simulink model "TP1_SIM_R3FOC_ctrl"  (R2023b)
settings: Solver=ode15s  StartTime=0.0  StopTime=0.2  FixedStep=1e-6  RelTol=1e-5  EnableMultiTasking=on
values from neighbouring files (symbols this model uses):
  deltat = deltat_2    (= 35)    [tp1_b.m]
  theta = 3    [tp1_b.m]
libraries: spsThyristorLib x6, spsNeutralLib x5, spsVoltageMeasurementLib x4, spsMeanLib x3, spsCurrentMeasurementLib x1, spsGroundLib x1, spsSeriesRLCLoadLib x1, spsThreePhaseProgrammableVoltageSourceLib x1, spspowerguiLib x1
settings Model: Creator=Monina  LastModifiedBy=Amadeo
settings SolverCC: AlgebraicLoopSolver=TrustRegion
settings DataIOCC: SaveFormat=Array  SignalLoggingSaveFormat=ModelDataLogs  ReturnWorkspaceOutputs=off
settings OptimizationCC: ExpressionDepthLimit=2147483647  LifeSpan=inf
settings DebuggingCC: UnderspecifiedInitializationDetection=Classic  MergeDetectMultiDrivingBlocksExec=none  SolverPrmCheckMsg=warning  FcnCallInpInsideContextMsg=warning  UnconnectedInputMsg=warning  UnconnectedOutputMsg=warning  UnconnectedLineMsg=warning  StateNameClashWarn=warning  SFUnexpectedBacktrackingDiag=warning  SFNoUnconditionalDefaultTransitionDiag=warning  SFExecutionAtInitializationDiag=none  ArithmeticOperatorsInVariantConditions=warning
settings HardwareCC: ProdBitPerPointer=32  ProdBitPerSizeT=32  ProdBitPerPtrDiffT=32  ProdLargestAtomicFloat=None  ProdIntDivRoundTo=Undefined  ProdEndianess=Unspecified  ProdWordSize=32  ProdHWDeviceType=32-bit Generic
settings ModelReferenceCC: EnableRefExpFcnMdlSchedulingChecks=on  PropagateSignalLabelsOutOfModel=off
settings SFSimCC: SimUseLocalCustomCode=off  CustomCodeUndefinedFunction=UseInterfaceOnly
settings RTWCC: RTWUseLocalCustomCode=off
settings CodeAppCC: StateflowObjectComments=on
settings GRTTargetCC: TargetLangStandard=C89/C90 (ANSI)  CombineOutputUpdateFcns=off  GRTInterface=on
settings ConfigComp: CovMetricSettings=dw  CovSaveCumulativeToWorkspaceVar=on  CovSaveSingleToWorkspaceVar=on  CovExternalEMLEnable=off  CovSFcnEnable=off
settings SimscapeCC: SimscapeNormalizeSystem=off

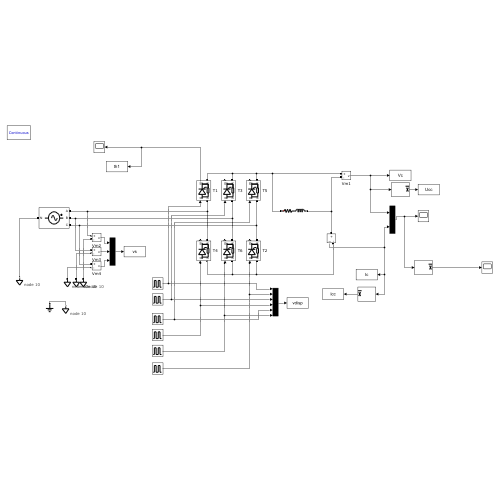
[thumbnail: Simulink's stored preview of the top-level diagram]
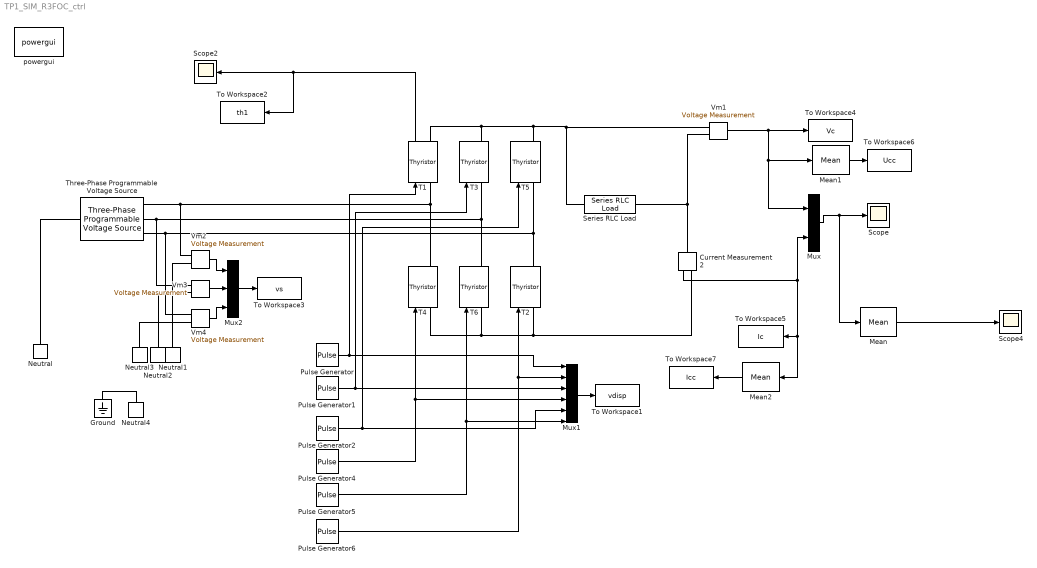
== system TP1_SIM_R3FOC_ctrl ==
  Current Measurement2 : spsCurrentMeasurementLib/Current Measurement  PhasorSimulation=off  OutputType=Complex  PSBequivalent=0
  Ground : spsGroundLib/Ground  LConnTagsString=a
  Mean : spsMeanLib/Mean  Freq=50  Vinit=0  Ts=0
  Mean1 : spsMeanLib/Mean  Freq=50  Vinit=0  Ts=0
  Mean2 : spsMeanLib/Mean  Freq=50  Vinit=0  Ts=0
  Mux : Mux  Inputs=2
  Mux1 : Mux  Inputs=6
  Mux2 : Mux  Inputs=3
  Neutral{,1..4} (5 alike) : spsNeutralLib/Neutral  LConnTagsString=a  NodeNumber=10
      settings: AttributesFormatString=node %<NodeNumber>  LibrarySourceBlock=sps_lib/Utilities/Neutral
  Pulse Generator : DiscretePulseGenerator  PulseType=Time based  Period=.02  PulseWidth=deltat  PhaseDelay=t(theta,1)
  Pulse Generator1 : DiscretePulseGenerator  PulseType=Time based  Period=.02  PulseWidth=deltat  PhaseDelay=t(theta,3)
  Pulse Generator2 : DiscretePulseGenerator  PulseType=Time based  Period=.02  PulseWidth=deltat  PhaseDelay=t(theta,5)
  Pulse Generator4 : DiscretePulseGenerator  PulseType=Time based  Period=.02  PulseWidth=deltat  PhaseDelay=t(theta,4)
  Pulse Generator5 : DiscretePulseGenerator  PulseType=Time based  Period=.02  PulseWidth=deltat  PhaseDelay=t(theta,6)
  Pulse Generator6 : DiscretePulseGenerator  PulseType=Time based  Period=.02  PulseWidth=deltat  PhaseDelay=t(theta,2)
  Scope : Scope
  Scope2 : Scope
  Scope4 : Scope
  Series RLC Load : spsSeriesRLCLoadLib/Series RLC Load  LConnTagsString=a  RConnTagsString=__new0  NominalVoltage=220  NominalFrequency=50  ActivePower=P  InductivePower=Q  CapacitivePower=0  Setx0=off  InitialVoltage=0  SetiL0=off  InitialCurrent=0  Measurements=None  LoadType=constant Z
  T{1..6} (6 alike) : spsThyristorLib/Thyristor  Ron=0.001  Lon=0  Vf=0.8  IC=0  Rs=400  Cs=500e-10  Measurements=on
  Three-Phase Programmable Voltage Source : spsThreePhaseProgrammableVoltageSourceLib/Three-Phase Programmable Voltage Source  PositiveSequence="[380  0 50]"  VariationEntity=None  VariationType=Table of time-amplitude pairs  VariationTypeAlt=Step  VariationStep=0.5  VariationRate=10  VariationMagnitude=0.3  VariationFrequency=2  VariationTiming=[1 2]  VariationPhaseA=off  Amplitudes=[1 0.8 1.2 1.0]  TimeValues=[0 0.1 0.15 0.2]  HarmonicGeneration=off  HarmonicA=[3 0.2 -25 0]  HarmonicB=[2 0.15 35 2]  Timing="[0.05  3]"  BusType=swing  Pref=0  Qref=0  Qmin=-inf  Qmax=inf
  To Workspace1 : ToWorkspace  VariableName=vdisp  SampleTime=-1
  To Workspace2 : ToWorkspace  VariableName=th1  SampleTime=-1
  To Workspace3 : ToWorkspace  VariableName=vs  SampleTime=-1
  To Workspace4 : ToWorkspace  VariableName=Vc  SampleTime=-1
  To Workspace5 : ToWorkspace  VariableName=Ic  SampleTime=-1
  To Workspace6 : ToWorkspace  VariableName=Ucc  SampleTime=-1
  To Workspace7 : ToWorkspace  VariableName=Icc  SampleTime=-1
  Vm{1..4} (4 alike) : spsVoltageMeasurementLib/Voltage Measurement  PhasorSimulation=off  OutputType=Complex  PSBequivalent=0
  powergui : spspowerguiLib/powergui  Priority=1  SimulationMode=Continuous  SampleTime=50e-6  frequency=60  Iterations=50  frequencyindice=50  Pbase=100e6  ErrMax=1e-4  UnitsV=kV  UnitsW=MW  buscounter=0  FunctionMessages=off  echomessages=off  EnableUseOfTLC=off  CurrentSourceSwitches=on  DisableSnubberDevices=off  DisableRonSwitches=off  DisableVfSwitches=off  DisplayEquations=off  AutomaticDiscreteSolvers=off  SolverType=Tustin  Interpol=off  ExternalGateDelay=off  methode=off  Ts=0  x0status=blocks  SPID=off  SwTol=0  HookPort=off  NonlinearTolerance=1e-4  nMaxIteration=100  ContinueOnMaxIteration=off  RestoreLinks=warning  ResistiveCurrentMeasurement=off  Frange=[0:2:500]  Ylog=off  Xlog=on  ShowGrid=off  save=off  variable=ZData  structure=0  ZoomFFT=off  StartTime=0.0  cycles=1  DisplayStyle=1  fundamental=60  FreqAxis=off  MaxFrequency=1000  frequencyindicesteady=1  RmsSteady=1  display=off
  wires:
  Mux/1 -> Mean/1, Scope/1
  T1/1 -> To Workspace2/1, Scope2/1
  Current Measurement2/1 -> Mean2/1, To Workspace5/1, Mux/2
  Pulse Generator1/1 -> Mux1/3, T3/1
  Vm2/1 -> Mux2/1
  Vm3/1 -> Mux2/2
  Vm4/1 -> Mux2/3
  Mux2/1 -> To Workspace3/1
  Vm1/1 -> To Workspace4/1, Mean1/1, Mux/1
  Mean/1 -> Scope4/1
  Pulse Generator4/1 -> Mux1/4, T4/1
  Pulse Generator6/1 -> T2/1, Mux1/2
  Mean1/1 -> To Workspace6/1
  Mean2/1 -> To Workspace7/1
  Pulse Generator5/1 -> Mux1/6, T6/1
  Pulse Generator/1 -> T1/1, Mux1/1
  Pulse Generator2/1 -> Mux1/5, T5/1
  Mux1/1 -> To Workspace1/1
  connections:
  Three-Phase Programmable Voltage Source/LConn1 -- Neutral/LConn1
  Series RLC Load/LConn1 -- Vm1/LConn1 -- T1/RConn1 -- T3/RConn1 -- T5/RConn1
  Current Measurement2/RConn1 -- T4/LConn1 -- T6/LConn1 -- T2/LConn1
  Current Measurement2/LConn1 -- Vm1/LConn2 -- Series RLC Load/RConn1
  Three-Phase Programmable Voltage Source/RConn2 -- Vm3/LConn1 -- T3/LConn1 -- T6/RConn1
  Three-Phase Programmable Voltage Source/RConn3 -- Vm4/LConn1 -- T5/LConn1 -- T2/RConn1
  T4/RConn1 -- Vm2/LConn1 -- Three-Phase Programmable Voltage Source/RConn1 -- T1/LConn1
  Vm2/LConn2 -- Neutral1/LConn1
  Neutral2/LConn1 -- Vm3/LConn2
  Vm4/LConn2 -- Neutral3/LConn1
  Neutral4/LConn1 -- Ground/LConn1
